simulink model "BLDC_system_diagram"  (R2013a)
settings: Solver=ode45  StartTime=0.0  StopTime=0.5  RelTol=1e-3
undefined symbols (not defined in the file or in its folder): Accelerationmax, Accelerationmin, DiscIntNeverNeededParam, IDCmax, IDCmin, Iphasepeakmax, P, PM, Risetimemax, Speedmax, Stalltimemax, Temperaturemax, Ts, VDCmax, VDCmin, VDCrated
undefined symbols (not defined in the file): Rs
libraries: simulink x68, powerlib_meascontrol x9, spsPMSynchronousMachineModel x3, simulink_extras x2
(part 2 of 3)

== system BLDC_system_diagram/Measurement System/Vdq0 Calculator ==
  note: =
  note: [Vd]
      | [Vq]
  note: [Valpha]
      | [Vbeta]
  note: [cos(wt)   sin(wt)]
      | [-sin(wt)  cos(wt)]
  note: [Va]
      | [Vb]
      | [Vc]
  note: [Valpha]
      | [Vbeta]
      | [V0]
  note: =(2/3)
  note: [   1                  -1/2              -1/2]
      | [      0       sqrt(3)/2     -sqrt(3)/2  ]
      | [    1/2              1/2             1/2   ]
  VABC : Inport
  Thetae : Inport  Port=2
  abc to dq1 : powerlib_meascontrol/Transformations/abc to dq0  Alignment=Aligned with phase A axis
  Vdq0 : Outport
  wires:
  abc to dq1/1 -> Vdq0/1
  Thetae/1 -> abc to dq1/2
  VABC/1 -> abc to dq1/1

== system BLDC_system_diagram/Open Loop Controller/Open Loop Controller ==
  note: void writestate (int sa, int sb, int sc)
      | {
      |   if (sa==1)    {digitalWrite(PhaseaUpperPin, HIGH);digitalWrite(PhaseaLowerPin, LOW);}
      |   if (sa==(-1)){digitalWrite(PhaseaUpperPin, LOW) ;digitalWrite(PhaseaLowerPin, HIGH);}
      |   if (sa==0)    {digitalWrite(PhaseaUpperPin, LOW) ;digitalWrite(PhaseaLowerPin, LOW);}
      |   if (sb==1)    {digitalWrite(PhasebUpperPin, HIGH);digitalWrite(PhasebLowerPin, LOW);}
      |   if (sb==(-1)){digitalWrite(PhasebUpperPin, LOW) ;digitalWrite(PhasebLowerPin, HIGH);}
      |   if (sb==0)    {digitalWrite(PhasebUpperPin, LOW) ;digitalWrite(PhasebLowerPin, LOW);}
      |   if (sc==1)    {digitalWrite(PhasecUpperPin, HIGH);digitalWrite(PhasecLowerPin, LOW);}
      |   if (sc==(-1)){digitalWrite(PhasecUpperPin, LOW) ;digitalWrite(PhasecLowerPin, HIGH);}
      |   if (sc==0)    {digitalWrite(PhasecUpperPin, LOW) ;digitalWrite(PhasecLowerPin, LOW);}
      | }
      |
      | void loop()
      | {
      |   HALLA=digitalRead(HallaPin);
      |   HALLB=digitalRead(HallbPin);
      |   HALLC=digitalRead(HallcPin);
      |   newstate=(HALLC<<2)|(HALLB<<1)|(HALLA);
      |
      | if (newstate==B000){writestate(0,0,0);}
      | if (newstate==B001){writestate(0,-1,1);}
      | if (newstate==B010){writestate(-1,1,0);}
      | if (newstate==B011){writestate(-1,0,1);}
      | if (newstate==B100){writestate(1,0,-1);}
      | if (newstate==B101){writestate(1,-1,0);}
      | if (newstate==B110){writestate(0,1,-1);}
      | if (newstate==B111){writestate(0,0,0);}
      | }
  note: Direction              EMF_ABC
      | 1(clockwise)           emf_abc
      | -1(anticlockwise)      -emf_abc
  HALLSensorABCSignals : Inport
  Direction : Inport  Port=2
  Decoder : Subsystem
  Gain : Gain  Gain=-1
  Gates : Subsystem
  Switch : Switch
  Gatings : Outport
  wires:
  Gates/1(Gates) -> Gatings/1
  Decoder/1(emf_abc) -> Switch/1, Gain/1
  HALLSensorABCSignals/1 -> Decoder/1("Hall ")
  Gain/1 -> Switch/3
  Direction/1 -> Switch/2
  Switch/1 -> Gates/1("emf_abc ")

== system BLDC_system_diagram/PWM Speed and Current Controller/PWM Speed and Current Controller ==
  note: void writestate (int sa, int sb, int sc)
      | {
      |   if (sa==1)    {digitalWrite(PhaseaUpperPin, HIGH);digitalWrite(PhaseaLowerPin, LOW);}
      |   if (sa==(-1)){digitalWrite(PhaseaUpperPin, LOW) ;digitalWrite(PhaseaLowerPin, HIGH);}
      |   if (sa==0)    {digitalWrite(PhaseaUpperPin, LOW) ;digitalWrite(PhaseaLowerPin, LOW);}
      |   if (sb==1)    {digitalWrite(PhasebUpperPin, HIGH);digitalWrite(PhasebLowerPin, LOW);}
      |   if (sb==(-1)){digitalWrite(PhasebUpperPin, LOW) ;digitalWrite(PhasebLowerPin, HIGH);}
      |   if (sb==0)    {digitalWrite(PhasebUpperPin, LOW) ;digitalWrite(PhasebLowerPin, LOW);}
      |   if (sc==1)    {digitalWrite(PhasecUpperPin, HIGH);digitalWrite(PhasecLowerPin, LOW);}
      |   if (sc==(-1)){digitalWrite(PhasecUpperPin, LOW) ;digitalWrite(PhasecLowerPin, HIGH);}
      |   if (sc==0)    {digitalWrite(PhasecUpperPin, LOW) ;digitalWrite(PhasecLowerPin, LOW);}
      | }
      |
      | void loop()
      | {
      |
      | if (abs(VTriangle+slope*Ts)<Vmax)
      | {
      | Vtriangle= VTriangle+slope*Ts;
      | }
      | else
      | {
      | slope=-slope;
      | Vtriangle= VTriangle+slope*Ts;
      | }
      |
      |   SpeedErrorOld=SpeedErrorNew;
      |   SpeedErrorNew=newspeed-Speedref;
      |   Currentref=kps*SpeedErrorNew+kis*(0.5)*(SpeedErrorNew+SpeedErrorOld)*Ts;
      |
      |   Current=analogRead(CurrentPin);
      |   CurrentErrorOld=CurrentErrorNew;
      |   CurrentErrorNew=Current-Currentref;
      |   Vref=kpc*CurrentErrorNew+kic*(0.5)*(CurrentErrorNew+CurrentErrorOld)*Ts;
      |
      |   if(Vref>Vtriangle){OpAmpOutput=1;}
      |   else{OpAmpOutput=0; }
      |   if (OpAmpOutput>0) {
      | if (newstate==B000){writestate(0,0,0);}
      | if (newstate==B001){writestate(0,-1,1);}
      | if (newstate==B010){writestate(-1,1,0);}
      | if (newstate==B011){writestate(-1,0,1);}
      | if (newstate==B100){writestate(1,0,-1);}
      | if (newstate==B101){writestate(1,-1,0);}
      | if (newstate==B110){writestate(0,1,-1);}
      | if (newstate==B111){writestate(0,0,0);}
      |   }
      |   else{writestate(0,0,0);}
      |
      |   delayMicroseconds(Ts);
      |
      | }
  note: Desired
      | Direction
      | 1 Clockwise
      | -1 Anticlockwise
  HALLABC : Inport
  IDCInput : Inport  Port=2
  RotorSpeed(rpm) : Inport  Port=3
  ReferenceRotorSpeed(rpm) : Inport  Port=4
  Abs : Abs
  Compare To Zero : simulink/Logic and Bit Operations/Compare To Zero  relop=>=  OutDataTypeStr=boolean
  Decoder : Subsystem
  Gain : Gain  Gain=-1
  Gates : Subsystem
  PID Controller : simulink/Continuous/PID Controller  Controller=PID  TimeDomain=Continuous-time  SampleTime=1  IntegratorMethod=Forward Euler  FilterMethod=Forward Euler  Form=Parallel  P=0.1  I=0.1  D=0  N=100  InitialConditionSource=internal  InitialConditionForIntegrator=0  InitialConditionForFilter=0  ExternalReset=none  LimitOutput=on  UpperSaturationLimit=100  LowerSaturationLimit=-100  LinearizeAsGain=on  AntiWindupMode=none  Kb=1  TrackingMode=off  Kt=1  PParamMin=[]  PParamMax=[]  IParamMin=[]  IParamMax=[]  DParamMin=[]  DParamMax=[]  NParamMin=[]  NParamMax=[]  KbParamMin=[]  KbParamMax=[]  KtParamMin=[]  KtParamMax=[]  POutMin=[]  POutMax=[]  IOutMin=[]  IOutMax=[]  DOutMin=[]  DOutMax=[]  NOutMin=[]  NOutMax=[]  KbOutMin=[]  KbOutMax=[]  KtOutMin=[]  KtOutMax=[]  IntegratorOutMin=[]  IntegratorOutMax=[]  FilterOutMin=[]  FilterOutMax=[]  SumOutMin=[]  SumOutMax=[]  SumI1OutMin=[]  SumI1OutMax=[]  SumI2OutMin=[]  SumI2OutMax=[]  SumI3OutMin=[]  SumI3OutMax=[]  SumDOutMin=[]  SumDOutMax=[]  SaturationOutMin=[]  SaturationOutMax=[]  IntegratorContinuousStateAttributes=''  IntegratorStateMustResolveToSignalObject=off  IntegratorRTWStateStorageClass=Auto  FilterContinuousStateAttributes=''  FilterStateMustResolveToSignalObject=off  FilterRTWStateStorageClass=Auto
  PID Controller1 : simulink/Continuous/PID Controller  Controller=PID  TimeDomain=Continuous-time  SampleTime=1  IntegratorMethod=Forward Euler  FilterMethod=Forward Euler  Form=Parallel  P=0.1  I=0.1  D=0  N=100  InitialConditionSource=internal  InitialConditionForIntegrator=0  InitialConditionForFilter=0  ExternalReset=none  LimitOutput=on  UpperSaturationLimit=0.99  LowerSaturationLimit=-0.99  LinearizeAsGain=on  AntiWindupMode=none  Kb=1  TrackingMode=off  Kt=1  PParamMin=[]  PParamMax=[]  IParamMin=[]  IParamMax=[]  DParamMin=[]  DParamMax=[]  NParamMin=[]  NParamMax=[]  KbParamMin=[]  KbParamMax=[]  KtParamMin=[]  KtParamMax=[]  POutMin=[]  POutMax=[]  IOutMin=[]  IOutMax=[]  DOutMin=[]  DOutMax=[]  NOutMin=[]  NOutMax=[]  KbOutMin=[]  KbOutMax=[]  KtOutMin=[]  KtOutMax=[]  IntegratorOutMin=[]  IntegratorOutMax=[]  FilterOutMin=[]  FilterOutMax=[]  SumOutMin=[]  SumOutMax=[]  SumI1OutMin=[]  SumI1OutMax=[]  SumI2OutMin=[]  SumI2OutMax=[]  SumI3OutMin=[]  SumI3OutMax=[]  SumDOutMin=[]  SumDOutMax=[]  SaturationOutMin=[]  SaturationOutMax=[]  IntegratorContinuousStateAttributes=''  IntegratorStateMustResolveToSignalObject=off  IntegratorRTWStateStorageClass=Auto  FilterContinuousStateAttributes=''  FilterStateMustResolveToSignalObject=off  FilterRTWStateStorageClass=Auto
  Product : Product
  Subsystem : Subsystem
  Sum : Sum  Inputs=|+-
  Sum1 : Sum  Inputs=|+-
  Sum2 : Sum  Inputs=|+-
  Switch : Switch  Criteria=u2 > Threshold
  TRI : powerlib_meascontrol/Pulse & Signal Generators/Triangle Generator  Freq=1e4  Phase=90  Ts=0
  Gatings : Outport
  wires:
  Sum/1 -> PID Controller/1
  PID Controller/1 -> Sum1/1
  HALLABC/1 -> Decoder/1("Hall ")
  RotorSpeed(rpm)/1 -> Product/2
  Gates/1(Gates) -> Gatings/1
  Compare To Zero/1 -> Gates/2(PWM)
  Subsystem/1(Direction) -> Product/1, Switch/2
  Switch/1 -> Gates/1("emf_abc ")
  Abs/1 -> Sum/1
  Product/1 -> Sum/2
  Gain/1 -> Switch/3
  Sum1/1 -> PID Controller1/1
  TRI/1 -> Sum2/2
  ReferenceRotorSpeed(rpm)/1 -> Subsystem/1(Speed), Abs/1
  IDCInput/1 -> Sum1/2
  PID Controller1/1 -> Sum2/1
  Decoder/1(emf_abc) -> Gain/1, Switch/1
  Sum2/1 -> Compare To Zero/1

== system BLDC_system_diagram/Protection System/AC overcurrent Protection ==
  StatorIABC : Inport
  C5 : simulink/Logic and Bit Operations/Compare To Constant  relop=>=  const=Iphasepeakmax  OutDataTypeStr=boolean
  C7 : simulink/Logic and Bit Operations/Compare To Constant  relop=>=  const=Iphasepeakmax  OutDataTypeStr=boolean
  C8 : simulink/Logic and Bit Operations/Compare To Constant  relop=>=  const=Iphasepeakmax  OutDataTypeStr=boolean
  Demux : Demux  Outputs=3
  Logical Operator : Logic  Operator=OR  Inputs=3  AllPortsSameDT=off  OutDataTypeStr=boolean
  Out1 : Outport
  wires:
  C5/1 -> Logical Operator/1
  C8/1 -> Logical Operator/3
  C7/1 -> Logical Operator/2
  StatorIABC/1 -> Demux/1
  Demux/2 -> C7/1
  Demux/3 -> C8/1
  Demux/1 -> C5/1
  Logical Operator/1 -> Out1/1

== system BLDC_system_diagram/Protection System/DC Over//Undervoltage Protection ==
  VDC : Inport
  C1 : simulink/Logic and Bit Operations/Compare To Constant  relop=<=  const=VDCmin  OutDataTypeStr=boolean
  C2 : simulink/Logic and Bit Operations/Compare To Constant  relop=>=  const=VDCmax  OutDataTypeStr=boolean
  Logical Operator7 : Logic  Operator=OR  AllPortsSameDT=off  OutDataTypeStr=boolean
  Out1 : Outport
  wires:
  VDC/1 -> C2/1, C1/1
  Logical Operator7/1 -> Out1/1
  C1/1 -> Logical Operator7/1
  C2/1 -> Logical Operator7/2

== system BLDC_system_diagram/Protection System/DC overcurrent Protection ==
  IDCInput : Inport
  C10 : simulink/Logic and Bit Operations/Compare To Constant  relop=<=  const=IDCmin  OutDataTypeStr=boolean
  C3 : simulink/Logic and Bit Operations/Compare To Constant  relop=>=  const=IDCmax  OutDataTypeStr=boolean
  Logical Operator6 : Logic  Operator=OR  AllPortsSameDT=off  OutDataTypeStr=boolean
  Out1 : Outport
  wires:
  C10/1 -> Logical Operator6/1
  C3/1 -> Logical Operator6/2
  IDCInput/1 -> C3/1, C10/1
  Logical Operator6/1 -> Out1/1

== system BLDC_system_diagram/Protection System/Excessive Acceleration//Deceleration Protection ==
  Acceleration : Inport
  C6 : simulink/Logic and Bit Operations/Compare To Constant  relop=<=  const=Accelerationmin  OutDataTypeStr=boolean
  C9 : simulink/Logic and Bit Operations/Compare To Constant  relop=>=  const=Accelerationmax  OutDataTypeStr=boolean
  Logical Operator5 : Logic  Operator=OR  AllPortsSameDT=off  OutDataTypeStr=boolean
  Out1 : Outport
  wires:
  C9/1 -> Logical Operator5/2
  Acceleration/1 -> C9/1, C6/1
  Logical Operator5/1 -> Out1/1
  C6/1 -> Logical Operator5/1

== system BLDC_system_diagram/Protection System/MOSFET Failure Protection ==
  Gatings : Inport
  StatorVABC : Inport  Port=2
  C1 : simulink/Logic and Bit Operations/Compare To Constant  relop=>  const=0  OutDataTypeStr=boolean
  C11 : simulink/Logic and Bit Operations/Compare To Constant  relop=>  const=VDCrated/2  OutDataTypeStr=boolean
  C12 : simulink/Logic and Bit Operations/Compare To Constant  relop=>  const=VDCrated/2  OutDataTypeStr=boolean
  C13 : simulink/Logic and Bit Operations/Compare To Constant  relop=>  const=VDCrated/2  OutDataTypeStr=boolean
  C2 : simulink/Logic and Bit Operations/Compare To Constant  relop=>  const=0  OutDataTypeStr=boolean
  C3 : simulink/Logic and Bit Operations/Compare To Constant  relop=>  const=0  OutDataTypeStr=boolean
  Demux1 : Demux  Outputs=6
  Demux2 : Demux  Outputs=3
  Logical Operator1 : Logic  Operator=XOR  AllPortsSameDT=off  OutDataTypeStr=boolean
  Logical Operator2 : Logic  Operator=XOR  AllPortsSameDT=off  OutDataTypeStr=boolean
  Logical Operator3 : Logic  Operator=XOR  AllPortsSameDT=off  OutDataTypeStr=boolean
  Logical Operator4 : Logic  Operator=OR  Inputs=3  AllPortsSameDT=off  OutDataTypeStr=boolean
  Timer1 : Subsystem
  Timer2 : Subsystem
  Timer3 : Subsystem
  Out1 : Outport
  wires:
  Logical Operator3/1 -> Timer3/1(In1)
  Demux2/3 -> C13/1
  Logical Operator2/1 -> Timer2/1(In1)
  StatorVABC/1 -> Demux2/1
  Gatings/1 -> Demux1/1
  Demux1/3 -> C2/1
  Demux1/1 -> C1/1
  Demux1/5 -> C3/1
  Demux2/1 -> C11/1
  C13/1 -> Logical Operator3/2
  C11/1 -> Logical Operator1/2
  Demux2/2 -> C12/1
  Logical Operator1/1 -> Timer1/1(In1)
  C12/1 -> Logical Operator2/2
  Logical Operator4/1 -> Out1/1
  C1/1 -> Logical Operator1/1
  C2/1 -> Logical Operator2/1
  C3/1 -> Logical Operator3/1
  Timer1/1(Out1) -> Logical Operator4/1
  Timer2/1(Out1) -> Logical Operator4/2
  Timer3/1(Out1) -> Logical Operator4/3

== system BLDC_system_diagram/Protection System/Overheating Protection ==
  Temperature : Inport
  C19 : simulink/Logic and Bit Operations/Compare To Constant  relop=>=  const=Temperaturemax  OutDataTypeStr=boolean
  Out1 : Outport
  wires:
  Temperature/1 -> C19/1
  C19/1 -> Out1/1

== system BLDC_system_diagram/Protection System/Overspeed and Stall Protection ==
  Speed(rpm) : Inport
  Add2 : Sum  Inputs=+-
  C17 : simulink/Logic and Bit Operations/Compare To Constant  relop===  const=0  OutDataTypeStr=boolean
  C18 : simulink/Logic and Bit Operations/Compare To Constant  relop=>=  const=Stalltimemax  OutDataTypeStr=boolean
  C4 : simulink/Logic and Bit Operations/Compare To Constant  relop=>=  const=Speedmax  OutDataTypeStr=boolean
  Clock : Clock
      settings: Decimation=1000000
  Edge Detector : powerlib_meascontrol/Logic/Edge Detector  model=Rising  ic=0  Ts=0
  Logical Operator8 : Logic  Operator=OR  AllPortsSameDT=off  OutDataTypeStr=boolean
  Switch : Switch  Criteria=u2 > Threshold
  Out1 : Outport
  wires:
  C18/1 -> Logical Operator8/1
  Logical Operator8/1 -> Out1/1
  Speed(rpm)/1 -> C4/1, C17/1
  Add2/1 -> C18/1
  C17/1 -> Edge Detector/1
  Switch/1 -> Switch/3, Add2/2
  Edge Detector/1 -> Switch/2
  Clock/1 -> Add2/1, Switch/1
  C4/1 -> Logical Operator8/2

== system BLDC_system_diagram/SVPWM Speed Controller/SVPWM Speed Controller ==
  HALLABC : Inport
  RotorSpeed(rpm) : Inport  Port=2
  ReferenceRotorSpeed(rpm) : Inport  Port=3
  3phases sin generator : Subsystem  AncestorBlock=AC2DriveInternalModels/SVM generator/3phases sin generator
  Abs : Abs
  Add : Sum
  Add1 : Sum  Inputs=+-
  Compare To Constant : simulink/Logic and Bit Operations/Compare To Constant  relop=>=  const=10  OutDataTypeStr=boolean
  Constant : Constant  Value=0.5
  Decoder : Subsystem
  PID Controller : simulink/Continuous/PID Controller  Controller=PID  TimeDomain=Continuous-time  SampleTime=1  IntegratorMethod=Forward Euler  FilterMethod=Forward Euler  Form=Parallel  P=0.1  I=1  D=0  N=100  InitialConditionSource=internal  InitialConditionForIntegrator=0  InitialConditionForFilter=0  ExternalReset=none  LimitOutput=on  UpperSaturationLimit=48  LowerSaturationLimit=-48  LinearizeAsGain=on  AntiWindupMode=none  Kb=1  TrackingMode=off  Kt=1  PParamMin=[]  PParamMax=[]  IParamMin=[]  IParamMax=[]  DParamMin=[]  DParamMax=[]  NParamMin=[]  NParamMax=[]  KbParamMin=[]  KbParamMax=[]  KtParamMin=[]  KtParamMax=[]  POutMin=[]  POutMax=[]  IOutMin=[]  IOutMax=[]  DOutMin=[]  DOutMax=[]  NOutMin=[]  NOutMax=[]  KbOutMin=[]  KbOutMax=[]  KtOutMin=[]  KtOutMax=[]  IntegratorOutMin=[]  IntegratorOutMax=[]  FilterOutMin=[]  FilterOutMax=[]  SumOutMin=[]  SumOutMax=[]  SumI1OutMin=[]  SumI1OutMax=[]  SumI2OutMin=[]  SumI2OutMax=[]  SumI3OutMin=[]  SumI3OutMax=[]  SumDOutMin=[]  SumDOutMax=[]  SaturationOutMin=[]  SaturationOutMax=[]  IntegratorContinuousStateAttributes=''  IntegratorStateMustResolveToSignalObject=off  IntegratorRTWStateStorageClass=Auto  FilterContinuousStateAttributes=''  FilterStateMustResolveToSignalObject=off  FilterRTWStateStorageClass=Auto
  Pole Pairs : Gain  Gain=4
  Product1 : Product
  SVPWM : Subsystem  mask{Fs=10000, Fsampling=10000, Vbase=48, Vdc=48}
  Sum : Sum  Inputs=|+-
  Switch : Switch  Threshold=100
  rpm to radpersecond : Gain  Gain=pi/30
  Gatings : Outport
  wires:
  rpm to radpersecond/1 -> Pole Pairs/1
  ReferenceRotorSpeed(rpm)/1 -> Sum/1
  SVPWM/1(Gatings) -> Gatings/1
  HALLABC/1 -> Decoder/1("Hall ")
  Decoder/1(emf_abc) -> Product1/2
  PID Controller/1 -> 3phases sin generator/2(Vcom), Product1/1  "V*"
  Switch/1 -> SVPWM/1(Vabc)
  Product1/1 -> Switch/3
  Sum/1 -> PID Controller/1, Compare To Constant/1
  Pole Pairs/1 -> Add/1
  3phases sin generator/1(Vabc) -> Switch/1
  RotorSpeed(rpm)/1 -> Abs/1, rpm to radpersecond/1, Sum/2
  Add/1 -> 3phases sin generator/1(Freq_com)
  Compare To Constant/1 -> Add1/1
  Add1/1 -> Add/2
  Constant/1 -> Add1/2
  Abs/1 -> Switch/2

== system BLDC_system_diagram/ Field Orinted ControlSVPWM Controller/ Field Orinted ControlSVPWM Controller/SVPWM ==
  Vabc : Inport
  Add : Sum
  Cartesian to Polar : simulink_extras/Transformations/Cartesian to Polar
  Constant : Constant  Value=2*pi
  Constant1 : Constant  Value=2*pi
  Constant2 : Constant  Value=Vdc
  Divide : Product  Inputs=/*
  Dwell Time Calculator : Subsystem
  Math Function : Math  Operator=rem  SaturateOnIntegerOverflow=on
  Pulses : Subsystem
  Saturation : Saturate  UpperLimit=0.99  LowerLimit=0  SampleTime=1/Fsampling
  Sector judge : Subsystem
  Ts : Constant  Value=1/Fs
  Unit Delay : UnitDelay  InitialCondition=1220  SampleTime=1/Fsampling
  Zero-Order Hold : ZeroOrderHold  SampleTime=1/(2*Fs)
  Zero-Order Hold1 : ZeroOrderHold  SampleTime=1/(2*Fs)
  abc/alphabeta : Subsystem
  constant : Gain  Gain=3^0.5
  constant2 : Gain  Gain=(1/Vbase)
  ma : Scope
      settings: SaveName=ScopeData5
  theta : Scope
      settings: YMin=-3.5  YMax=10  SaveName=ScopeData6
  Gatings : Outport
  wires:
  Dwell Time Calculator/3(T0) -> Pulses/4(T0)
  constant/1 -> Divide/2
  Pulses/1(Gating) -> Gatings/1
  Cartesian to Polar/1 -> constant/1
  Divide/1 -> Saturation/1
  Ts/1 -> Dwell Time Calculator/3(Ts)
  Dwell Time Calculator/1(Ta) -> Pulses/2(Ta1)
  Dwell Time Calculator/2(Tb) -> Pulses/3(Tb1)
  Sector judge/2(Cal_theta) -> Dwell Time Calculator/1(Theta)
  Saturation/1 -> Zero-Order Hold/1, ma/1
  Zero-Order Hold/1 -> Dwell Time Calculator/2(ma)
  Constant2/1 -> Divide/1
  Zero-Order Hold1/1 -> Sector judge/1(theta), theta/1
  Sector judge/1(Sector) -> Pulses/1(Sector)
  abc/alphabeta/1(Valpha) -> Cartesian to Polar/1
  abc/alphabeta/2(Vbeta) -> Cartesian to Polar/2
  Cartesian to Polar/2 -> Add/1
  Math Function/1 -> Zero-Order Hold1/1
  Constant/1 -> Add/2
  Add/1 -> Math Function/1
  Constant1/1 -> Math Function/2
  Vabc/1 -> abc/alphabeta/1(Vabc)

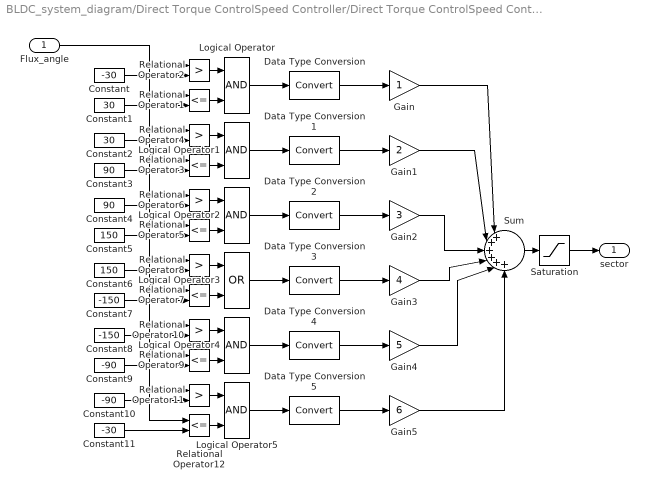
== system BLDC_system_diagram/Direct Torque ControlSpeed Controller/Direct Torque ControlSpeed Controller/Flux sector seeker ==
  Flux_angle : Inport
  Constant : Constant  Value=-30
  Constant1 : Constant  Value=30
  Constant10 : Constant  Value=-90
  Constant11 : Constant  Value=-30
  Constant2 : Constant  Value=30
  Constant3 : Constant  Value=90
  Constant4 : Constant  Value=90
  Constant5 : Constant  Value=150
  Constant6 : Constant  Value=150
  Constant7 : Constant  Value=-150
  Constant8 : Constant  Value=-150
  Constant9 : Constant  Value=-90
  Data Type Conversion{,1..5} (6 alike) : DataTypeConversion  SaturateOnIntegerOverflow=on  RndMeth=Zero
  Gain : Gain  SaturateOnIntegerOverflow=on  OutDataTypeStr=Inherit: Same as input  ParamDataTypeStr=Inherit: Same as input
  Gain1 : Gain  Gain=2  SaturateOnIntegerOverflow=on  OutDataTypeStr=Inherit: Same as input  ParamDataTypeStr=Inherit: Same as input
  Gain2 : Gain  Gain=3  SaturateOnIntegerOverflow=on  OutDataTypeStr=Inherit: Same as input  ParamDataTypeStr=Inherit: Same as input
  Gain3 : Gain  Gain=4  SaturateOnIntegerOverflow=on  OutDataTypeStr=Inherit: Same as input  ParamDataTypeStr=Inherit: Same as input
  Gain4 : Gain  Gain=5  SaturateOnIntegerOverflow=on  OutDataTypeStr=Inherit: Same as input  ParamDataTypeStr=Inherit: Same as input
  Gain5 : Gain  Gain=6  SaturateOnIntegerOverflow=on  OutDataTypeStr=Inherit: Same as input  ParamDataTypeStr=Inherit: Same as input
  Logical Operator{,1..2,4..5} (5 alike) : Logic
  Logical Operator3 : Logic  Operator=OR
  Relational Operator{1,3,5,7,9,12} (6 alike) : RelationalOperator  Operator=<=  InputSameDT=on
  Relational Operator{2,4,6,8,10..11} (6 alike) : RelationalOperator  Operator=>  InputSameDT=on
  Saturation : Saturate  UpperLimit=6  LowerLimit=1
  Sum : Sum  Inputs=|++++++  SaturateOnIntegerOverflow=on  InputSameDT=on  OutDataTypeStr=Inherit: Same as first input
  sector : Outport
  wires:
  Data Type Conversion5/1 -> Gain5/1
  Data Type Conversion4/1 -> Gain4/1
  Data Type Conversion3/1 -> Gain3/1
  Data Type Conversion2/1 -> Gain2/1
  Data Type Conversion1/1 -> Gain1/1
  Data Type Conversion/1 -> Gain/1
  Saturation/1 -> sector/1
  Sum/1 -> Saturation/1
  Gain5/1 -> Sum/6
  Gain4/1 -> Sum/5
  Gain3/1 -> Sum/4
  Gain2/1 -> Sum/3
  Gain1/1 -> Sum/2
  Gain/1 -> Sum/1
  Constant11/1 -> Relational Operator12/2
  Constant10/1 -> Relational Operator11/2
  Logical Operator5/1 -> Data Type Conversion5/1
  Relational Operator12/1 -> Logical Operator5/2
  Relational Operator11/1 -> Logical Operator5/1
  Constant9/1 -> Relational Operator9/2
  Constant8/1 -> Relational Operator10/2
  Logical Operator4/1 -> Data Type Conversion4/1
  Relational Operator9/1 -> Logical Operator4/2
  Relational Operator10/1 -> Logical Operator4/1
  Constant7/1 -> Relational Operator7/2
  Constant6/1 -> Relational Operator8/2
  Logical Operator3/1 -> Data Type Conversion3/1
  Relational Operator7/1 -> Logical Operator3/2
  Relational Operator8/1 -> Logical Operator3/1
  Constant5/1 -> Relational Operator5/2
  Constant4/1 -> Relational Operator6/2
  Logical Operator2/1 -> Data Type Conversion2/1
  Relational Operator5/1 -> Logical Operator2/2
  Relational Operator6/1 -> Logical Operator2/1
  Constant3/1 -> Relational Operator3/2
  Constant2/1 -> Relational Operator4/2
  Logical Operator1/1 -> Data Type Conversion1/1
  Relational Operator3/1 -> Logical Operator1/2
  Relational Operator4/1 -> Logical Operator1/1
  Constant1/1 -> Relational Operator1/2
  Constant/1 -> Relational Operator2/2
  Flux_angle/1 -> Relational Operator12/1, Relational Operator11/1, Relational Operator9/1, Relational Operator10/1, Relational Operator7/1, Relational Operator8/1, Relational Operator5/1, Relational Operator6/1, Relational Operator3/1, Relational Operator4/1, Relational Operator1/1, Relational Operator2/1
  Logical Operator/1 -> Data Type Conversion/1
  Relational Operator1/1 -> Logical Operator/2
  Relational Operator2/1 -> Logical Operator/1

== system BLDC_system_diagram/Direct Torque ControlSpeed Controller/Direct Torque ControlSpeed Controller/Flux table ==
  |N| : Inport
  Abs1 : Abs  SaturateOnIntegerOverflow=on
  F : Fcn  Expr=bs*nf/u(1)
  Saturation : Saturate  UpperLimit=inf  LowerLimit=bs
  Flux : Outport
  wires:
  Abs1/1 -> Saturation/1
  F/1 -> Flux/1
  |N|/1 -> Abs1/1
  Saturation/1 -> F/1

== system BLDC_system_diagram/Direct Torque ControlSpeed Controller/Direct Torque ControlSpeed Controller/Switching table ==
  H Te : Inport
  H Phi : Inport  Port=2
  Sector : Inport  Port=3
  Constant1 : Constant
  Flux = -1 : Lookup2D  RowIndex=[1;2;3]  ColumnIndex=[1;2;3;4;5;6]  Table=[3 4 5 6 1 2;7 0 7 0 7 0;5 6 1 2 3 4]  SaturateOnIntegerOverflow=on
  Flux = 1 : Lookup2D  RowIndex=[1;2;3]  ColumnIndex=[1;2;3;4;5;6]  Table=[2 3 4 5 6 1;0 7 0 7 0 7;6 1 2 3 4 5]  SaturateOnIntegerOverflow=on
  Multiport Switch1 : MultiPortSwitch  Inputs=2  SaturateOnIntegerOverflow=on
  Multiport Switch2 : MultiPortSwitch  Inputs=8  SaturateOnIntegerOverflow=on
  Scope1 : Scope
      settings: YMin=-1  YMax=10  SaveName=ScopeData4
  Sum1 : Sum  Inputs=|++  SaturateOnIntegerOverflow=on
  v0 : Constant  Value=[0 1 0 1 0 1]
  v1 : Constant  Value=[1 0 0 1 0 1]
  v2 : Constant  Value=[1 0 1 0 0 1]
  v3 : Constant  Value=[0 1 1 0 0 1]
  v4 : Constant  Value=[0 1 1 0 1 0]
  v5 : Constant  Value=[0 1 0 1 1 0]
  v6 : Constant  Value=[1 0 0 1 1 0]
  v7 : Constant  Value=[1 0 1 0 1 0]
  Gates : Outport
  wires:
  Multiport Switch2/1 -> Gates/1
  v5/1 -> Multiport Switch2/7
  v3/1 -> Multiport Switch2/5
  v6/1 -> Multiport Switch2/8
  v2/1 -> Multiport Switch2/4
  Multiport Switch1/1 -> Sum1/1
  Sum1/1 -> Scope1/1, Multiport Switch2/1
  Constant1/1 -> Sum1/2
  Flux = -1/1 -> Multiport Switch1/3
  Flux = 1/1 -> Multiport Switch1/2
  H Phi/1 -> Multiport Switch1/1
  Sector/1 -> Flux = 1/2, Flux = -1/2
  v7/1 -> Multiport Switch2/9
  v4/1 -> Multiport Switch2/6
  v1/1 -> Multiport Switch2/3
  v0/1 -> Multiport Switch2/2
  H Te/1 -> Flux = 1/1, Flux = -1/1

== system BLDC_system_diagram/Direct Torque ControlSpeed Controller/Direct Torque ControlSpeed Controller/Torque & Flux calculator ==
  V_abc : Inport
  I_ABC : Inport  Port=2
  Complex to Magnitude-Angle : ComplexToMagnitudeAngle
  Gain : Gain  Gain=Rss  SaturateOnIntegerOverflow=on  OutDataTypeStr=Inherit: Same as input  ParamDataTypeStr=Inherit: Same as input
  Gain1 : Gain  Gain=Rss  SaturateOnIntegerOverflow=on  OutDataTypeStr=Inherit: Same as input  ParamDataTypeStr=Inherit: Same as input
  Gain2 : Gain  Gain=3/2*P  SaturateOnIntegerOverflow=on  OutDataTypeStr=Inherit: Same as input  ParamDataTypeStr=Inherit: Same as input
  Gain5 : Gain  Gain=-1  SaturateOnIntegerOverflow=on  OutDataTypeStr=Inherit: Same as input  ParamDataTypeStr=Inherit: Same as input
  Product : Product  SaturateOnIntegerOverflow=on  OutDataTypeStr=Inherit: Same as first input
  Product1 : Product  SaturateOnIntegerOverflow=on  OutDataTypeStr=Inherit: Same as first input
  Rad2Deg : Gain  Gain=180/pi  SaturateOnIntegerOverflow=on  OutDataTypeStr=Inherit: Same as input  ParamDataTypeStr=Inherit: Same as input
  Real-Imag to Complex : RealImagToComplex
  Sum : Sum  Inputs=|+-  SaturateOnIntegerOverflow=on
  Sum1 : Sum  Inputs=|+-  SaturateOnIntegerOverflow=on
  Sum3 : Sum  Inputs=-+  SaturateOnIntegerOverflow=on
  Zero-Order Hold1 : ZeroOrderHold  SampleTime=Ts
  Zero-Order Hold2 : ZeroOrderHold  SampleTime=Ts
  Zero-Order Hold3 : ZeroOrderHold  SampleTime=Ts
  dq_I_transform : Subsystem
  dq_V_transform : Subsystem
  phi_d : DiscreteIntegrator  IntegratorMethod=Integration: Trapezoidal  SampleTime=Ts  ICPrevOutput=DiscIntNeverNeededParam  ICPrevScaledInput=DiscIntNeverNeededParam
  phi_q : DiscreteIntegrator  IntegratorMethod=Integration: Trapezoidal  SampleTime=Ts  ICPrevOutput=DiscIntNeverNeededParam  ICPrevScaledInput=DiscIntNeverNeededParam
  Torque : Outport
  Flux : Outport  Port=2
  angle : Outport  Port=3
  wires:
  Zero-Order Hold3/1 -> angle/1
  Zero-Order Hold1/1 -> Flux/1
  Zero-Order Hold2/1 -> Torque/1
  Product1/1 -> Sum3/2
  Gain5/1 -> Real-Imag to Complex/2
  Rad2Deg/1 -> Zero-Order Hold3/1
  Complex to Magnitude-Angle/2 -> Rad2Deg/1
  Complex to Magnitude-Angle/1 -> Zero-Order Hold1/1
  Real-Imag to Complex/1 -> Complex to Magnitude-Angle/1
  I_ABC/1 -> dq_I_transform/1(I_abc)
  V_abc/1 -> dq_V_transform/1(Vabc)
  dq_V_transform/1(v_q) -> Sum/1
  dq_I_transform/1(I_q) -> Gain/1, Product1/2  "i_qs"
  Gain/1 -> Sum/2
  Sum/1 -> phi_q/1
  dq_V_transform/2(v_d) -> Sum1/1
  Gain1/1 -> Sum1/2
  dq_I_transform/2(I_d) -> Product/2, Gain1/1  "i_ds"
  Sum1/1 -> phi_d/1
  phi_q/1 -> Real-Imag to Complex/1, Product/1
  phi_d/1 -> Product1/1, Gain5/1
  Product/1 -> Sum3/1
  Sum3/1 -> Gain2/1
  Gain2/1 -> Zero-Order Hold2/1

== system BLDC_system_diagram/Field Oriented Controller/Field Oriented Control Current and Speed Controller/Current Controller ==
  Iabc_ref : Inport
  Iabc : Inport  Port=2
  BusCreator : BusCreator  Inputs=6
  Data Type Conversion{1..6} (6 alike) : DataTypeConversion  SaturateOnIntegerOverflow=on  RndMeth=Zero
  Demux : Demux  Outputs=3
  Demux3 : Demux  Outputs=3
  Logical Operator1 : Logic  Operator=NOT
  Logical Operator2 : Logic  Operator=NOT
  Logical Operator3 : Logic  Operator=NOT
  Relay : Relay  OnSwitchValue=1/2  OffSwitchValue=-1/2
  Relay4 : Relay  OnSwitchValue=1/2  OffSwitchValue=-1/2
  Relay5 : Relay  OnSwitchValue=1/2  OffSwitchValue=-1/2
  Sum4 : Sum  Inputs=-+  SaturateOnIntegerOverflow=on  InputSameDT=on  OutDataTypeStr=Inherit: Same as first input
  Sum5 : Sum  Inputs=-+  SaturateOnIntegerOverflow=on  InputSameDT=on  OutDataTypeStr=Inherit: Same as first input
  Sum6 : Sum  Inputs=-+  SaturateOnIntegerOverflow=on  InputSameDT=on  OutDataTypeStr=Inherit: Same as first input
  Pulses : Outport
  wires:
  Iabc/1 -> Demux3/1
  Demux/2 -> Sum5/2
  Demux/1 -> Sum4/2
  Sum4/1 -> Relay/1
  Demux3/2 -> Sum5/1
  Demux3/1 -> Sum4/1
  Sum5/1 -> Relay4/1
  Demux3/3 -> Sum6/1
  Demux/3 -> Sum6/2
  Sum6/1 -> Relay5/1
  Iabc_ref/1 -> Demux/1
  Logical Operator2/1 -> Data Type Conversion4/1
  Data Type Conversion5/1 -> Logical Operator2/1
  Relay/1 -> BusCreator/1, Data Type Conversion5/1
  Data Type Conversion4/1 -> BusCreator/2
  Logical Operator1/1 -> Data Type Conversion1/1
  Data Type Conversion2/1 -> Logical Operator1/1
  Data Type Conversion1/1 -> BusCreator/4
  Logical Operator3/1 -> Data Type Conversion3/1
  Data Type Conversion6/1 -> Logical Operator3/1
  Data Type Conversion3/1 -> BusCreator/6
  Relay4/1 -> BusCreator/3, Data Type Conversion2/1
  Relay5/1 -> BusCreator/5, Data Type Conversion6/1
  BusCreator/1 -> Pulses/1

== system BLDC_system_diagram/Hysteresis Speed and Current Controller/Hysteresis Speed and Current Controller/Current Controller ==
  Iabc_ref : Inport
  Iabc : Inport  Port=2
  BusCreator : BusCreator  Inputs=6
  Data Type Conversion{1..6} (6 alike) : DataTypeConversion  SaturateOnIntegerOverflow=on  RndMeth=Zero
  Demux : Demux  Outputs=3
  Demux3 : Demux  Outputs=3
  Logical Operator1 : Logic  Operator=NOT
  Logical Operator2 : Logic  Operator=NOT
  Logical Operator3 : Logic  Operator=NOT
  Relay : Relay  OnSwitchValue=1/2  OffSwitchValue=-1/2
  Relay4 : Relay  OnSwitchValue=1/2  OffSwitchValue=-1/2
  Relay5 : Relay  OnSwitchValue=1/2  OffSwitchValue=-1/2
  Sum4 : Sum  Inputs=-+  SaturateOnIntegerOverflow=on  InputSameDT=on  OutDataTypeStr=Inherit: Same as first input
  Sum5 : Sum  Inputs=-+  SaturateOnIntegerOverflow=on  InputSameDT=on  OutDataTypeStr=Inherit: Same as first input
  Sum6 : Sum  Inputs=-+  SaturateOnIntegerOverflow=on  InputSameDT=on  OutDataTypeStr=Inherit: Same as first input
  Pulses : Outport
  wires:
  Iabc/1 -> Demux3/1
  Demux/2 -> Sum5/2
  Demux/1 -> Sum4/2
  Sum4/1 -> Relay/1
  Demux3/2 -> Sum5/1
  Demux3/1 -> Sum4/1
  Sum5/1 -> Relay4/1
  Demux3/3 -> Sum6/1
  Demux/3 -> Sum6/2
  Sum6/1 -> Relay5/1
  Iabc_ref/1 -> Demux/1
  Logical Operator2/1 -> Data Type Conversion4/1
  Data Type Conversion5/1 -> Logical Operator2/1
  Relay/1 -> BusCreator/1, Data Type Conversion5/1
  Data Type Conversion4/1 -> BusCreator/2
  Logical Operator1/1 -> Data Type Conversion1/1
  Data Type Conversion2/1 -> Logical Operator1/1
  Data Type Conversion1/1 -> BusCreator/4
  Logical Operator3/1 -> Data Type Conversion3/1
  Data Type Conversion6/1 -> Logical Operator3/1
  Data Type Conversion3/1 -> BusCreator/6
  Relay4/1 -> BusCreator/3, Data Type Conversion2/1
  Relay5/1 -> BusCreator/5, Data Type Conversion6/1
  BusCreator/1 -> Pulses/1

== system BLDC_system_diagram/Hysteresis Speed and Current Controller/Hysteresis Speed and Current Controller/Decoder ==
  note: This module implements the following true table
      |
      |    ha   |   hb   |   hc   ||   emf_a   |   emf_b   |   emf_c
      |     --------------------------------------------------------------------------------
      | 0          0         0          0               0               0
      | 0          0         1          0               -1              +1
      | 0          1         0          -1              +1                0
      | 0          1         1          -1               0               +1
      | 1          0         0         +1               0               -1
      | 1          0         1         +1              -1                0
      | 1          1         0          0              +1               -1
      | 1          1         1          0               0                0
  note: ha
  note: /hc
  note: hc
  note: /hb
  note: hb
  note: /ha
  note: /ha
  note: hc
  note: /hc
  note: hb
  note: /hb
  note: ha
  note: ha
  note: /ha
  "Hall " : Inport
  Data Type Conversion{1..6} (6 alike) : DataTypeConversion
  Demux1 : Demux  Outputs=3
  Demux2 : Demux  Outputs=3
  Logical Operator1 : Logic  Operator=NOT  AllPortsSameDT=off  OutDataTypeStr=boolean
  Logical Operator{2..7} (6 alike) : Logic  AllPortsSameDT=off  OutDataTypeStr=boolean
  Mux1 : Mux  Inputs=3
  Sum1 : Sum  Inputs=+-  OutDataTypeStr=double
  Sum2 : Sum  Inputs=+-  OutDataTypeStr=double
  Sum3 : Sum  Inputs=+-  OutDataTypeStr=double
  Hall_abc : Outport
  wires:
  Data Type Conversion6/1 -> Sum3/2
  Data Type Conversion3/1 -> Sum3/1
  Data Type Conversion4/1 -> Sum2/2
  Data Type Conversion1/1 -> Sum1/1
  Logical Operator7/1 -> Data Type Conversion6/1
  Logical Operator5/1 -> Data Type Conversion4/1
  Data Type Conversion2/1 -> Sum2/1
  Logical Operator4/1 -> Data Type Conversion3/1
  Logical Operator3/1 -> Data Type Conversion1/1
  Mux1/1 -> Hall_abc/1
  Sum3/1 -> Mux1/3
  Sum1/1 -> Mux1/2
  Sum2/1 -> Mux1/1
  Logical Operator2/1 -> Data Type Conversion2/1
  Demux1/2 -> Logical Operator6/1, Logical Operator2/2
  Demux1/3 -> Logical Operator7/1, Logical Operator3/2
  Demux2/1 -> Logical Operator7/2, Logical Operator2/1
  Data Type Conversion5/1 -> Sum1/2
  Demux1/1 -> Logical Operator5/1, Logical Operator4/2
  Demux2/2 -> Logical Operator5/2, Logical Operator3/1
  Logical Operator6/1 -> Data Type Conversion5/1
  Demux2/3 -> Logical Operator6/2, Logical Operator4/1
  "Hall "/1 -> Demux2/1, Logical Operator1/1
  Logical Operator1/1 -> Demux1/1

== system BLDC_system_diagram/Measurement System/Speed, Acceleration, Direction and Angles Calculator/Acceleration Calculator ==
  note: Acceleration=dSpeed/dt
      | dt=Ts=Sampling Time
  Speed : Inport
  Add : Sum  Inputs=+-
  Constant : Constant  Value=Ts
  Divide : Product  Inputs=*/
  Sampler : ZeroOrderHold  SampleTime=Ts
  Acceleration : Outport
  wires:
  Speed/1 -> Add/1, Sampler/1
  Sampler/1 -> Add/2
  Add/1 -> Divide/1
  Constant/1 -> Divide/2
  Divide/1 -> Acceleration/1

== system BLDC_system_diagram/Measurement System/Speed, Acceleration, Direction and Angles Calculator/Clock and Direction ==
  note: Change Detected when oldThetae
      | is not equal to new Thetae
      |
      | Direction                                                                                               Change
      | 1 (clockwise)                       always positive except when cycle is completed (-4*(pi/3))
      | -1 (anticlockwise)                 always negative except when cycle is completed (4*(pi/3))
  Change Detected : Inport
  Add3 : Sum  Inputs=-+-+  OutDataTypeStr=double
  C1 : simulink/Logic and Bit Operations/Compare To Constant  relop=>=  const=240*(pi/180)  OutDataTypeStr=boolean
  C2 : simulink/Logic and Bit Operations/Compare To Constant  relop=<=  const=-240*(pi/180)  OutDataTypeStr=boolean
  C3 : simulink/Logic and Bit Operations/Compare To Zero  relop=<  OutDataTypeStr=boolean
  C4 : simulink/Logic and Bit Operations/Compare To Zero  relop=>  OutDataTypeStr=boolean
  C5 : simulink/Logic and Bit Operations/Compare To Zero  relop===  OutDataTypeStr=boolean
  Gain7 : Gain  Gain=2
  Gain8 : Gain  Gain=2
  NOT : Logic  Operator=NOT  AllPortsSameDT=off  OutDataTypeStr=boolean
  Scope2 : Scope
      settings: YMin=-7  YMax=7  SaveName=ScopeData11
  Switch2 : Switch  Criteria=u2 > Threshold
  Direction : Outport
  Clock : Outport  Port=2
  wires:
  Change Detected/1 -> Scope2/1, C5/1, C2/1, C1/1, C4/1, C3/1
  C3/1 -> Add3/1
  C5/1 -> NOT/1
  Add3/1 -> Switch2/1
  Gain7/1 -> Add3/3
  Gain8/1 -> Add3/4
  NOT/1 -> Switch2/2, Clock/1
  C4/1 -> Add3/2
  C1/1 -> Gain7/1
  C2/1 -> Gain8/1
  Switch2/1 -> Switch2/3, Direction/1

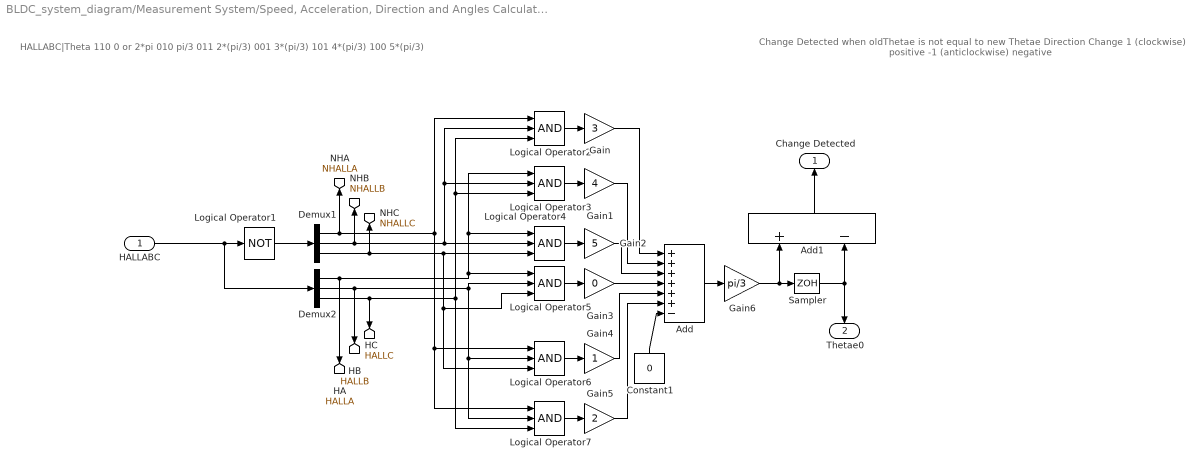
== system BLDC_system_diagram/Measurement System/Speed, Acceleration, Direction and Angles Calculator/HALL change Detector ==
  note: Change Detected when oldThetae
      | is not equal to new Thetae
      |
      | Direction                         Change
      | 1 (clockwise)                        positive
      | -1 (anticlockwise)                 negative
  note: HALLABC|Theta
      | 110    0 or 2*pi
      | 010           pi/3
      | 011     2*(pi/3)
      | 001      3*(pi/3)
      | 101      4*(pi/3)
      | 100     5*(pi/3)
  HALLABC : Inport
  Add : Sum  Inputs=++++++-
  Add1 : Sum  Inputs=+-
  Constant1 : Constant  Value=0
  Demux1 : Demux  Outputs=3
  Demux2 : Demux  Outputs=3
  Gain : Gain  Gain=3
  Gain1 : Gain  Gain=4
  Gain2 : Gain  Gain=5
  Gain3 : Gain  Gain=0
  Gain4 : Gain
  Gain5 : Gain  Gain=2
  Gain6 : Gain  Gain=pi/3  ParamDataTypeStr=double
  Logical Operator1 : Logic  Operator=NOT  AllPortsSameDT=off  OutDataTypeStr=boolean
  Logical Operator{2..7} (6 alike) : Logic  Inputs=3  AllPortsSameDT=off  OutDataTypeStr=boolean
  Sampler : ZeroOrderHold  SampleTime=1.01*Ts
  Change Detected : Outport
  Thetae0 : Outport  Port=2
  tag scope: HALLA=global, HALLB=global, HALLC=global, NHALLA=global, NHALLB=global, NHALLC=global
  wires:
  Logical Operator6/1 -> Gain4/1
  Gain/1 -> Add/1
  Logical Operator3/1 -> Gain1/1
  Gain1/1 -> Add/2
  Add1/1 -> Change Detected/1
  Add/1 -> Gain6/1
  Demux1/1 -> [NHALLA], Logical Operator7/1, Logical Operator6/1, Logical Operator2/1
  Gain2/1 -> Add/3
  Demux2/3 -> Logical Operator7/3, Logical Operator3/3, Logical Operator2/3, [HALLC]
  Demux2/1 -> [HALLA], Logical Operator4/1, Logical Operator3/1, Logical Operator5/1
  Logical Operator1/1 -> Demux1/1
  Logical Operator5/1 -> Gain3/1
  Demux1/2 -> Logical Operator3/2, Logical Operator2/2, Logical Operator4/2, [NHALLB]
  Demux2/2 -> Logical Operator6/2, Logical Operator7/2, Logical Operator5/2, [HALLB]
  Gain4/1 -> Add/5
  Logical Operator4/1 -> Gain2/1
  HALLABC/1 -> Logical Operator1/1, Demux2/1
  Gain6/1 -> Add1/1, Sampler/1
  Gain5/1 -> Add/6
  Logical Operator7/1 -> Gain5/1
  Logical Operator2/1 -> Gain/1
  Gain3/1 -> Add/4
  Demux1/3 -> Logical Operator6/3, Logical Operator5/3, Logical Operator4/3, [NHALLC]
  Sampler/1 -> Thetae0/1, Add1/2
  Constant1/1 -> Add/7

== system BLDC_system_diagram/Measurement System/Speed, Acceleration, Direction and Angles Calculator/Speed Calculator ==
  note: dTheta=pi/3
      | ElectricalSpeed(rad/s)=(dThetae/dt)*Direction
      | ElectricalSpeed(rpm)=ElectricalSpeed(rad/s)*(30/pi)
      | MechanicalSpeed(rpm)=ElectricalSpeed(rpm)/PolePairs
      | P=Pole Pairs=Poles/2
  Clk : Inport
  Add2 : Sum  Inputs=-+
  Avoid Division by zero : Switch  Criteria=u2 > Threshold
  Clock : Clock
      settings: Decimation=1000000
  Compare To Zero : simulink/Logic and Bit Operations/Compare To Zero  relop=>  OutDataTypeStr=boolean
  Constant1 : Constant  Value=((pi/3)*60)/(P*(2*pi))
  Divide : Product  Inputs=*/*  LockScale=on
  Edge Detector : powerlib_meascontrol/Logic/Edge Detector  model=Falling  ic=0  Ts=-1
  Speed (rpm) : Scope
      settings: YMin=-5000  YMax=5000  SaveName=ScopeData8
  Switch : Switch  Criteria=u2 > Threshold
  Switch1 : Switch  Criteria=u2 > Threshold
  Speed : Outport
  New Clock Time : Outport  Port=2
  Old Clock Time : Outport  Port=3
  wires:
  Clk/1 -> Edge Detector/1, Switch1/2
  Divide/1 -> Avoid Division by zero/1
  Constant1/1 -> Divide/1
  Clock/1 -> Switch/1
  Switch1/1 -> Old Clock Time/1, Switch1/3, Add2/1
  [Direction] -> Divide/3
  Add2/1 -> Compare To Zero/1, Divide/2
  Edge Detector/1 -> Switch/2
  Switch/1 -> Add2/2, New Clock Time/1, Switch/3, Switch1/1
  Compare To Zero/1 -> Avoid Division by zero/2
  Avoid Division by zero/1 -> Speed/1, Speed (rpm)/1, Avoid Division by zero/3

== system BLDC_system_diagram/Measurement System/Speed, Acceleration, Direction and Angles Calculator/Subsystem ==
  note: Thetae=Theta0+dTheta
      | Case                                 Thetae
      | 0<=Thetae<=(2*pi)           Thetae
      | Thetae<0                 2*pi+Thetae
      | Thetae>(2*pi)           Thetae-2*pi
  Theta0 : Inport
  dTheta : Inport  Port=2
  Add : Sum
  Add1 : Sum
  Add2 : Sum  Inputs=+-
  Add3 : Sum  Inputs=+++
  CC : simulink/Logic and Bit Operations/Compare To Constant  relop=<  const=0  OutDataTypeStr=boolean
  CC1 : simulink/Logic and Bit Operations/Compare To Constant  relop=>  const=2*pi  OutDataTypeStr=boolean
  CC2 : simulink/Logic and Bit Operations/Compare To Constant  relop=>=  const=0  OutDataTypeStr=boolean
  CC3 : simulink/Logic and Bit Operations/Compare To Constant  relop=<=  const=2*pi  OutDataTypeStr=boolean
  Constant : Constant  Value=2*pi
  Constant1 : Constant  Value=2*pi
  Gain : Gain  Gain=2
  Gain1 : Gain  Gain=3
  Logical Operator : Logic  AllPortsSameDT=off  OutDataTypeStr=boolean
  Multiport Switch : MultiPortSwitch
  Thetae : Outport
  wires:
  Theta0/1 -> Add1/1
  dTheta/1 -> Add1/2
  Constant1/1 -> Add2/2
  Constant/1 -> Add/2
  Add2/1 -> Multiport Switch/4
  Multiport Switch/1 -> Thetae/1
  Add/1 -> Multiport Switch/3
  CC/1 -> Gain/1
  CC1/1 -> Gain1/1
  CC3/1 -> Logical Operator/1
  CC2/1 -> Logical Operator/2
  Add3/1 -> Multiport Switch/1
  Gain1/1 -> Add3/3
  Gain/1 -> Add3/2
  Logical Operator/1 -> Add3/1
  Add1/1 -> CC2/1, CC3/1, CC/1, CC1/1, Add2/1, Multiport Switch/2, Add/1

== system BLDC_system_diagram/Measurement System/Speed, Acceleration, Direction and Angles Calculator/delta Thetae Calculator ==
  note: dThetae=Speed*dt
      | dt=Time since last change of Thetae / HALL signals
  Speed (rpm) : Inport
  Last Clock Time : Inport  Port=2
  Add : Sum  Inputs=+-
  Current Time : Clock
      settings: Decimation=1000000
  Gain : Gain  Gain=(P*2*pi)/60
  Product : Product
  dThetae : Outport
  wires:
  Last Clock Time/1 -> Add/2
  Current Time/1 -> Add/1
  Gain/1 -> Product/2
  Product/1 -> dThetae/1
  Add/1 -> Product/1
  Speed (rpm)/1 -> Gain/1

== system BLDC_system_diagram/Measurement System/Torque & Flux calculator/dq_I_transform ==
  I_ab : Inport
  Demux : Demux  Outputs=2
  Gain : Gain  Gain=1/2  SaturateOnIntegerOverflow=on  OutDataTypeStr=Inherit: Same as input  ParamDataTypeStr=Inherit: Same as input
  Gain1 : Gain  Gain=1/2  SaturateOnIntegerOverflow=on  OutDataTypeStr=Inherit: Same as input  ParamDataTypeStr=Inherit: Same as input
  Gain2 : Gain  Gain=2/3  SaturateOnIntegerOverflow=on  OutDataTypeStr=Inherit: Same as input  ParamDataTypeStr=Inherit: Same as input
  Gain3 : Gain  Gain=sqrt(3)/2  SaturateOnIntegerOverflow=on  OutDataTypeStr=Inherit: Same as input  ParamDataTypeStr=Inherit: Same as input
  Gain4 : Gain  Gain=sqrt(3)/2  SaturateOnIntegerOverflow=on  OutDataTypeStr=Inherit: Same as input  ParamDataTypeStr=Inherit: Same as input
  Gain5 : Gain  Gain=2/3  SaturateOnIntegerOverflow=on  OutDataTypeStr=Inherit: Same as input  ParamDataTypeStr=Inherit: Same as input
  Sum2 : Sum  Inputs=-+  SaturateOnIntegerOverflow=on  InputSameDT=on  OutDataTypeStr=Inherit: Same as first input
  Sum3 : Sum  Inputs=+--  SaturateOnIntegerOverflow=on  InputSameDT=on  OutDataTypeStr=Inherit: Same as first input
  Sum4 : Sum  Inputs=--  SaturateOnIntegerOverflow=on  InputSameDT=on  OutDataTypeStr=Inherit: Same as first input
  I_q : Outport
  I_d : Outport  Port=2
  wires:
  Sum2/1 -> Gain5/1
  Gain4/1 -> Sum2/2
  Gain3/1 -> Sum2/1
  Sum3/1 -> Gain2/1
  Sum4/1 -> Gain4/1, Gain1/1
  Gain/1 -> Sum3/2
  Gain1/1 -> Sum3/3
  Demux/2 -> Sum4/2, Gain/1, Gain3/1
  Demux/1 -> Sum4/1, Sum3/1
  I_ab/1 -> Demux/1
  Gain5/1 -> I_d/1
  Gain2/1 -> I_q/1

== system BLDC_system_diagram/Measurement System/Torque & Flux calculator/dq_V_transform ==
  Vabc : Inport
  Demux : Demux  Outputs=3
  Gain : Gain  Gain=1/2  SaturateOnIntegerOverflow=on  OutDataTypeStr=Inherit: Same as input  ParamDataTypeStr=Inherit: Same as input
  Gain1 : Gain  Gain=1/2  SaturateOnIntegerOverflow=on  OutDataTypeStr=Inherit: Same as input  ParamDataTypeStr=Inherit: Same as input
  Gain2 : Gain  Gain=2/3  SaturateOnIntegerOverflow=on  OutDataTypeStr=Inherit: Same as input  ParamDataTypeStr=Inherit: Same as input
  Gain3 : Gain  Gain=sqrt(3)/2  SaturateOnIntegerOverflow=on  OutDataTypeStr=Inherit: Same as input  ParamDataTypeStr=Inherit: Same as input
  Gain4 : Gain  Gain=sqrt(3)/2  SaturateOnIntegerOverflow=on  OutDataTypeStr=Inherit: Same as input  ParamDataTypeStr=Inherit: Same as input
  Gain5 : Gain  Gain=2/3  SaturateOnIntegerOverflow=on  OutDataTypeStr=Inherit: Same as input  ParamDataTypeStr=Inherit: Same as input
  Sum2 : Sum  Inputs=+--  SaturateOnIntegerOverflow=on  InputSameDT=on  OutDataTypeStr=Inherit: Same as first input
  Sum3 : Sum  Inputs=-+  SaturateOnIntegerOverflow=on  InputSameDT=on  OutDataTypeStr=Inherit: Same as first input
  v_q : Outport
  v_d : Outport  Port=2
  wires:
  Sum3/1 -> Gain5/1
  Gain4/1 -> Sum3/2
  Gain3/1 -> Sum3/1
  Gain2/1 -> v_q/1
  Gain1/1 -> Sum2/3
  Gain/1 -> Sum2/2
  Demux/1 -> Sum2/1
  Sum2/1 -> Gain2/1
  Gain5/1 -> v_d/1
  Vabc/1 -> Demux/1
  Demux/2 -> Gain/1, Gain3/1
  Demux/3 -> Gain1/1, Gain4/1

== system BLDC_system_diagram/Open Loop Controller/Open Loop Controller/Decoder ==
  note: /ha
  note: ha
  note: ha
  note: /hb
  note: hb
  note: /hc
  note: hc
  note: /ha
  note: /ha
  note: hb
  note: /hb
  note: hc
  note: /hc
  note: ha
  note: This module implements the following true table
      |
      |    ha   |   hb   |   hc   ||   emf_a   |   emf_b   |   emf_c
      |     --------------------------------------------------------------------------------
      | 0          0         0          0               0               0
      | 0          0         1          0               -1              +1
      | 0          1         0          -1              +1                0
      | 0          1         1          -1               0               +1
      | 1          0         0         +1               0               -1
      | 1          0         1         +1              -1                0
      | 1          1         0          0              +1               -1
      | 1          1         1          0               0                0
  "Hall " : Inport
  Data Type Conversion{1..6} (6 alike) : DataTypeConversion
  Demux1 : Demux  Outputs=3
  Demux2 : Demux  Outputs=3
  Logical Operator1 : Logic  Operator=NOT  AllPortsSameDT=off  OutDataTypeStr=boolean
  Logical Operator{2..7} (6 alike) : Logic  AllPortsSameDT=off  OutDataTypeStr=boolean
  Mux1 : Mux  Inputs=3
  Sum1 : Sum  Inputs=+-  OutDataTypeStr=double
  Sum2 : Sum  Inputs=+-  OutDataTypeStr=double
  Sum3 : Sum  Inputs=+-  OutDataTypeStr=double
  emf_abc : Outport
  wires:
  "Hall "/1 -> Logical Operator1/1, Demux2/1
  Logical Operator1/1 -> Demux1/1
  Demux2/3 -> Logical Operator4/1, Logical Operator6/2
  Demux2/2 -> Logical Operator3/1, Logical Operator5/2
  Demux2/1 -> Logical Operator2/1, Logical Operator7/2
  Demux1/3 -> Logical Operator3/2, Logical Operator7/1
  Demux1/2 -> Logical Operator2/2, Logical Operator6/1
  Demux1/1 -> Logical Operator4/2, Logical Operator5/1
  Logical Operator2/1 -> Data Type Conversion2/1
  Sum2/1 -> Mux1/1
  Sum1/1 -> Mux1/2
  Sum3/1 -> Mux1/3
  Mux1/1 -> emf_abc/1
  Logical Operator3/1 -> Data Type Conversion1/1
  Logical Operator4/1 -> Data Type Conversion3/1
  Logical Operator5/1 -> Data Type Conversion4/1
  Logical Operator6/1 -> Data Type Conversion5/1
  Logical Operator7/1 -> Data Type Conversion6/1
  Data Type Conversion2/1 -> Sum2/1
  Data Type Conversion4/1 -> Sum2/2
  Data Type Conversion1/1 -> Sum1/1
  Data Type Conversion5/1 -> Sum1/2
  Data Type Conversion3/1 -> Sum3/1
  Data Type Conversion6/1 -> Sum3/2

== system BLDC_system_diagram/Open Loop Controller/Open Loop Controller/Gates ==
  note: This module implements the following true table
      |
      |    emf_a   |   emf_b   |   emf_c   ||   Q1   |   Q2   |   Q3   |   Q4   |   Q5   |   Q6
      |     ------------------------------------------------------------------------------------------------------------------
      |       0              0                0            0          0          0           0        0        0
      |       0               -1              +1          0          0          0           1        1        0
      |     -1              +1                0          0          1          1           0        0        0
      |     -1               0               +1          0          1         0           0        1        0
      |    +1               0                -1          1          0          0           0        0        1
      |    +1              -1                0           1          0          0           1        0        0
      |      0              +1               -1           0          0          1           0        0        1
      |     0              0                0             0          0          0           0        0        0
  "emf_abc " : Inport
  Compare To Zero : simulink/Logic and Bit Operations/Compare To Zero  relop=>  OutDataTypeStr=boolean  ZeroCross=off
  Compare To Zero1 : simulink/Logic and Bit Operations/Compare To Zero  relop=<  OutDataTypeStr=boolean  ZeroCross=off
  Compare To Zero2 : simulink/Logic and Bit Operations/Compare To Zero  relop=>  OutDataTypeStr=boolean  ZeroCross=off
  Compare To Zero3 : simulink/Logic and Bit Operations/Compare To Zero  relop=<  OutDataTypeStr=boolean  ZeroCross=off
  Compare To Zero4 : simulink/Logic and Bit Operations/Compare To Zero  relop=>  OutDataTypeStr=boolean  ZeroCross=off
  Compare To Zero5 : simulink/Logic and Bit Operations/Compare To Zero  relop=<  OutDataTypeStr=boolean  ZeroCross=off
  Demux2 : Demux  Outputs=3
  Mux3 : Mux  Inputs=6
  Gates : Outport
  wires:
  "emf_abc "/1 -> Demux2/1
  Mux3/1 -> Gates/1
  Demux2/1 -> Compare To Zero/1, Compare To Zero1/1
  Demux2/2 -> Compare To Zero2/1, Compare To Zero3/1
  Demux2/3 -> Compare To Zero4/1, Compare To Zero5/1
  Compare To Zero/1 -> Mux3/1
  Compare To Zero1/1 -> Mux3/2
  Compare To Zero2/1 -> Mux3/3
  Compare To Zero3/1 -> Mux3/4
  Compare To Zero4/1 -> Mux3/5
  Compare To Zero5/1 -> Mux3/6

== system BLDC_system_diagram/PWM Speed and Current Controller/PWM Speed and Current Controller/Decoder ==
  note: /ha
  note: ha
  note: ha
  note: /hb
  note: hb
  note: /hc
  note: hc
  note: /ha
  note: /ha
  note: hb
  note: /hb
  note: hc
  note: /hc
  note: ha
  note: This module implements the following true table
      |
      |    ha   |   hb   |   hc   ||   emf_a   |   emf_b   |   emf_c
      |     --------------------------------------------------------------------------------
      | 0          0         0          0               0               0
      | 0          0         1          0               -1              +1
      | 0          1         0          -1              +1                0
      | 0          1         1          -1               0               +1
      | 1          0         0         +1               0               -1
      | 1          0         1         +1              -1                0
      | 1          1         0          0              +1               -1
      | 1          1         1          0               0                0
  "Hall " : Inport
  Data Type Conversion{1..6} (6 alike) : DataTypeConversion
  Demux1 : Demux  Outputs=3
  Demux2 : Demux  Outputs=3
  Logical Operator1 : Logic  Operator=NOT  AllPortsSameDT=off  OutDataTypeStr=boolean
  Logical Operator{2..7} (6 alike) : Logic  AllPortsSameDT=off  OutDataTypeStr=boolean
  Mux1 : Mux  Inputs=3
  Sum1 : Sum  Inputs=+-  OutDataTypeStr=double
  Sum2 : Sum  Inputs=+-  OutDataTypeStr=double
  Sum3 : Sum  Inputs=+-  OutDataTypeStr=double
  emf_abc : Outport
  wires:
  "Hall "/1 -> Logical Operator1/1, Demux2/1
  Logical Operator1/1 -> Demux1/1
  Demux2/3 -> Logical Operator4/1, Logical Operator6/2
  Demux2/2 -> Logical Operator3/1, Logical Operator5/2
  Demux2/1 -> Logical Operator2/1, Logical Operator7/2
  Demux1/3 -> Logical Operator3/2, Logical Operator7/1
  Demux1/2 -> Logical Operator2/2, Logical Operator6/1
  Demux1/1 -> Logical Operator4/2, Logical Operator5/1
  Logical Operator2/1 -> Data Type Conversion2/1
  Sum2/1 -> Mux1/1
  Sum1/1 -> Mux1/2
  Sum3/1 -> Mux1/3
  Mux1/1 -> emf_abc/1
  Logical Operator3/1 -> Data Type Conversion1/1
  Logical Operator4/1 -> Data Type Conversion3/1
  Logical Operator5/1 -> Data Type Conversion4/1
  Logical Operator6/1 -> Data Type Conversion5/1
  Logical Operator7/1 -> Data Type Conversion6/1
  Data Type Conversion2/1 -> Sum2/1
  Data Type Conversion4/1 -> Sum2/2
  Data Type Conversion1/1 -> Sum1/1
  Data Type Conversion5/1 -> Sum1/2
  Data Type Conversion3/1 -> Sum3/1
  Data Type Conversion6/1 -> Sum3/2
